simulink library "basic_create_EB"  (R2018b)
settings: Solver=ode45  StartTime=0.0  StopTime=10.0  RelTol=1e-3  EnableMultiTasking=on
libraries: carnot x3
settings Model: Creator=lena.frank  LastModifiedBy=P41573
settings DataIOCC: LimitDataPoints=on  SaveFormat=Array  SignalLoggingSaveFormat=ModelDataLogs
settings OptimizationCC: ExpressionDepthLimit=2147483647  LifeSpan=inf
settings DebuggingCC: UnderspecifiedInitializationDetection=Classic  MergeDetectMultiDrivingBlocksExec=none  SolverPrmCheckMsg=warning  FcnCallInpInsideContextMsg=warning  StateNameClashWarn=warning  SFUnexpectedBacktrackingDiag=warning  SFNoUnconditionalDefaultTransitionDiag=warning  SFExecutionAtInitializationDiag=none
settings HardwareCC: ProdBitPerPointer=32  ProdBitPerSizeT=32  ProdBitPerPtrDiffT=32  ProdLargestAtomicFloat=None  ProdIntDivRoundTo=Undefined  ProdEndianess=Unspecified  ProdWordSize=32  ProdHWDeviceType=32-bit Generic
settings ModelReferenceCC: PropagateSignalLabelsOutOfModel=off
settings SFSimCC: SimUseLocalCustomCode=off
settings RTWCC: RTWUseLocalCustomCode=off
settings CodeAppCC: StateflowObjectComments=on
settings GRTTargetCC: TargetLangStandard=C89/C90 (ANSI)  GeneratePreprocessorConditionals=Disable all  CombineOutputUpdateFcns=off  GRTInterface=on
settings ConfigComp: CovMetricSettings=dw  CovHtmlReporting=on  CovSaveCumulativeToWorkspaceVar=on  CovSaveSingleToWorkspaceVar=on  CovExternalEMLEnable=off

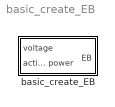
== system basic_create_EB ==
  basic_create_EB : Subsystem  InitFcn=load('EB.mat')  mask(basic_create_EB){eID=Power only, f=50, pf1=1, pf2=1, pf3=1}
      mask prompts: eID "ID for electric calculation"; f "frequency [Hz]"; pf1 "power factor line 1 [-]"; pf2 "power factor line 2 [-]"; pf3 "power factor line 3 [-]"
      mask help: Block to create an EB with the variable inputs ActPower and Voltage. The other values can be set as constants in the mask.
      mask Help: web(fullfile(path_carnot('help'),'basic_create_EB.html'),'-helpbrowser')
      mask TypeOptions eID: basic_EB/eID
      mask TypeOptions f: basic_EB/f
      mask TypeOptions pf1: basic_EB/pf1
      mask TypeOptions pf2: basic_EB/pf2
      mask TypeOptions pf3: basic_EB/pf3

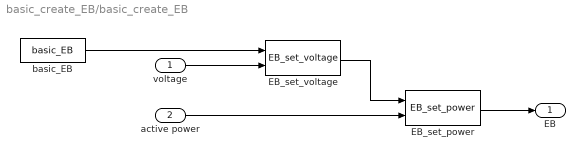
== system basic_create_EB/basic_create_EB ==
  voltage : Inport
  active power : Inport  Port=2
  EB_set_power : carnot/Source/Simple/EB_set_power
      settings: SourceProductName=Carnot
  EB_set_voltage : carnot/Source/Simple/EB_set_voltage
      settings: SourceProductName=Carnot
  basic_EB : carnot/Basic/Electric/basic_EB  eID=Power only  f=f  v1=230  p1=0  pf1=pf1  v2=230  p2=0  pf2=pf2  v3=230  p3=0  pf3=pf3
      settings: SourceProductName=Carnot
  EB : Outport
  wires:
  EB_set_voltage/1 -> EB_set_power/1
  basic_EB/1 -> EB_set_voltage/1
  active power/1 -> EB_set_power/2
  voltage/1 -> EB_set_voltage/2
  EB_set_power/1 -> EB/1
